simulink model "mcb_pmsm_hall_offset_f28035"  (R2021b)
settings: Solver=FixedStepDiscrete  StartTime=0.0  StopTime=Inf  RelTol=1e-3  EnableMultiTasking=on
InitFcn:
  | mcb_c2000_pmsm_offset_data;
  | target = mcb_SetProcessorDetails('F28035',PWM_frequency);
values from neighbouring files (symbols this model uses):
  PWM_frequency = 20e3    (= 20000)    [c28027pmsmfoc_data.m]    (also in c28035pmsmfoc_data.m; c28035pmsmfoc_data_cla.m = 12000; c28069pmsmfoc_data.m; mcb_c2000_open_loop_control_data.m = eval(get_param([bdroot '/Open Loop Control/Parameters/PWM Fr)
  Ts = 5e-8    (= 5e-08)    [DCDC_Buck_Param.m]    (also in mcb_c2000_open_loop_control_data.m = T_pwm; mcb_c2000_pmsm_offset_data.m = T_pwm; mcb_pmsm_foc_dual_f28379d_data.m = 5e-05; mcb_pmsm_foc_dual_f28379d_datascript.m = 5e-05)
undefined symbols (not defined in the file or in its folder): Down, GPTRIP1SEL, GPTRIP2SEL, motor, TZ1, TZ2, Up
libraries: idelinklib_common x14, simulink x5, mcbcontrolslib x5, mcbpositiondecoderlib x4, c2802xlib x4, c280xlib x3, hall_sensor_lib x3, c2803xlib x2, demo_controls x1, c2000lib x1
(part 2 of 2)

== system mcb_pmsm_hall_offset_f28035/Offset Calculation/Data Serial Output/While Iterator Subsystem ==
  Data : Inport
  Iteration : Inport  Port=2
  Add : Sum  Inputs=+-  OutDataTypeStr=Inherit: Same as first input
  Index Vector : MultiPortSwitch  Inputs=1
  SCI Transmit : c280xlib/SCI Transmit  sciModule=A  dataHead=''  dataTail=''  postInterrupt=off  numFifo=1
  While Iterator : WhileIterator  MaxIters=-1  WhileBlockType=do-while  ShowIterationPort=on  OutputDataType=int16
  wires:
  Iteration/1 -> Add/1
  Add/1 -> While Iterator/1
  Index Vector/1 -> SCI Transmit/1
  Data/1 -> Index Vector/2
  While Iterator/1 -> Index Vector/1, Add/2

== system mcb_pmsm_hall_offset_f28035/Offset Calculation/Subsystem/Calculate Position from Hall ==
  Calculate Counts : Subsystem  TreatAsAtomicUnit=on
  Data Store Read : DataStoreRead  DataStoreName=GlobalHallState  IndexOptions=Index vector (dialog)  Indices=1  OutputSizes=1
  Data Store Read2 : DataStoreRead  DataStoreName=GlobalSpeedCount  IndexOptions=Index vector (dialog)  Indices=1  OutputSizes=1
  Data Store Read3 : DataStoreRead  DataStoreName=GlobalDirection  IndexOptions=Index vector (dialog)  Indices=1  OutputSizes=1
  Data Store Read4 : DataStoreRead  DataStoreName=GlobalSpeedValidity  IndexOptions=Index vector (dialog)  Indices=1  OutputSizes=1
  Data Store Read5 : DataStoreRead  Priority=1  DataStoreName=HallStateChangeFlag  IndexOptions=Index vector (dialog)  Indices=1  OutputSizes=1
  Data Store Write2 : DataStoreWrite  Priority=2  DataStoreName=HallStateChangeFlag  IndexOptions=Index vector (dialog)  Indices=1  OutputSizes=1
  Hall Speed and Position : mcbpositiondecoderlib/Hall Speed and Position  blkExecutionType=Position  CounterSize=32 bits  ClkFreq=target.CPU_frequency  BlkSampleTime=Ts  PolePairs=motor.polePairs  MinSpeed=20  HallInterruptConfig=Every 180 Degrees  SpeedUnit=Per unit  PerUnitSpeed=6000  SpeedDataType=dataType  hallSequence=ABC  Sequence=[5,4,6,2,3,1]  EnableSecondOrder=1st Order  PositionUnit=Per unit  PositionDataType=dataType
      settings: SourceProductBaseCode=MT
  Pos_PU : Outport  InitialOutput=0  VectorParamsAs1DForOutWhenUnconnected=off
  wires:
  Hall Speed and Position/2 -> Data Store Write2/1
  Data Store Read/1 -> Calculate Counts/1(Halls), Hall Speed and Position/1
  Data Store Read5/1 -> Hall Speed and Position/6
  Data Store Read4/1 -> Hall Speed and Position/5
  Calculate Counts/1(Counter/Offset) -> Hall Speed and Position/2
  Data Store Read2/1 -> Hall Speed and Position/3
  Hall Speed and Position/1 -> Pos_PU/1
  Data Store Read3/1 -> Calculate Counts/2(Direction), Hall Speed and Position/4

== system mcb_pmsm_hall_offset_f28035/Offset Calculation/Control_System/Find Offset/Subsystem ==
  Theta_hall : Inport
  Enable : EnablePort
  IIR Filter : mcbcontrolslib/IIR Filter  VariantControl=Low Pass Filter  VariantSelect=Low-pass  Filter_constant=0.5  advancedSettings=off  Ts=50e-6  cutOff_freq=3183.0989
      settings: SourceProductBaseCode=MT
  Offset : Outport
  wires:
  IIR Filter/1 -> Offset/1
  Theta_hall/1 -> IIR Filter/1

== system mcb_pmsm_hall_offset_f28035/Offset Calculation/Control_System/PosGen/Subsystem ==
  Enable : EnablePort
  Constant : Constant  Value=0  OutDataTypeStr=Inherit: Inherit via back propagation
  Data Store Write : DataStoreWrite  DataStoreName=Enable  IndexOptions=Index vector (dialog)  Indices=1  OutputSizes=1
  wires:
  Constant/1 -> Data Store Write/1

== system mcb_pmsm_hall_offset_f28035/Offset Calculation/Control_System/PosGen/Subsystem1 ==
  Count : Inport
  Count for 2 sec : Constant  Value=2.5 * PWM_frequency  OutDataTypeStr=uint32  SampleTime=-1
  If : If  NumInputs=2  IfExpression=u1 < u2
  If Action Subsystem : Subsystem  TreatAsAtomicUnit=on
  If Action Subsystem2 : Subsystem  TreatAsAtomicUnit=on
  Merge : Merge
  Position Generator : mcbcontrolslib/Position Generator  AngleOutput=Per-unit  ThetaSource=External  ThetaInput=5e-4  DataType=double  ExternalReset=none  Offset=0
      settings: SourceProductBaseCode=MT
  Eps : Outport
  wires:
  If Action Subsystem/1(Out1) -> Merge/1
  If/1 -> If Action Subsystem/Action
  If Action Subsystem2/1(Out1) -> Merge/2
  Position Generator/1 -> Eps/1  "Eps"
  Count/1 -> If/1
  Merge/1 -> Position Generator/1
  If/2 -> If Action Subsystem2/Action
  Count for 2 sec/1 -> If/2

== system mcb_pmsm_hall_offset_f28035/Offset Calculation/Control_System/PosGen/Up Counter ==
  Enable : EnablePort  StatesWhenEnabling=reset
  Add1 : Sum  SaturateOnIntegerOverflow=on
  Constant : Constant  OutDataTypeStr=uint32
  Delay : Delay  DelayLength=1
  Count : Outport  OutputWhenDisabled=reset  InitialOutput=0
  wires:
  Add1/1 -> Count/1, Delay/1
  Constant/1 -> Add1/1
  Delay/1 -> Add1/2

== system mcb_pmsm_hall_offset_f28035/Offset Calculation/Subsystem/Calculate Position from Hall/Calculate Counts ==
  Halls : Inport
  Direction : Inport  Port=2
  Data Type Conversion2 : DataTypeConversion  OutDataTypeStr=uint32  ConvertRealWorld=Stored Integer (SI)
  Direction 0 Provides offset and counter values : Subsystem  TreatAsAtomicUnit=on
  Direction 1 Provides offset and counter values : Subsystem  TreatAsAtomicUnit=on
  Merge : Merge
  Switch on direction : If  IfExpression=u1 == 1
  Counter/Offset : Outport
  wires:
  Merge/1 -> Data Type Conversion2/1
  Switch on direction/2 -> Direction 1 Provides offset and counter values/Action
  Halls/1 -> Direction 0 Provides offset and counter values/1(halls), Direction 1 Provides offset and counter values/1(halls)
  Direction/1 -> Switch on direction/1
  Direction 0 Provides offset and counter values/1(counter) -> Merge/1
  Switch on direction/1 -> Direction 0 Provides offset and counter values/Action
  Direction 1 Provides offset and counter values/1(counter) -> Merge/2
  Data Type Conversion2/1 -> Counter/Offset/1

== system mcb_pmsm_hall_offset_f28035/Offset Calculation/Control_System/PosGen/Subsystem1/If Action Subsystem ==
  Action Port : ActionPort  ActionPortLabel=if(u1 < u2)
  Constant : Constant  Value=0  OutDataTypeStr=dataType
  Out1 : Outport
  wires:
  Constant/1 -> Out1/1

== system mcb_pmsm_hall_offset_f28035/Offset Calculation/Control_System/PosGen/Subsystem1/If Action Subsystem2 ==
  Action Port : ActionPort  ActionPortLabel=else
  Add1 : Sum
  Constant1 : Constant  Value=1e-3  OutDataTypeStr=dataType
  Delay : Delay  DelayLength=1
  Multiply : Gain  Gain=Ts  OutDataTypeStr=Inherit: Same as input
  Saturate to 60 RPM : Saturate  UpperLimit=motor.polePairs  LowerLimit=0
  Out1 : Outport
  wires:
  Delay/1 -> Add1/2
  Constant1/1 -> Add1/1
  Multiply/1 -> Out1/1
  Add1/1 -> Saturate to 60 RPM/1
  Saturate to 60 RPM/1 -> Multiply/1, Delay/1

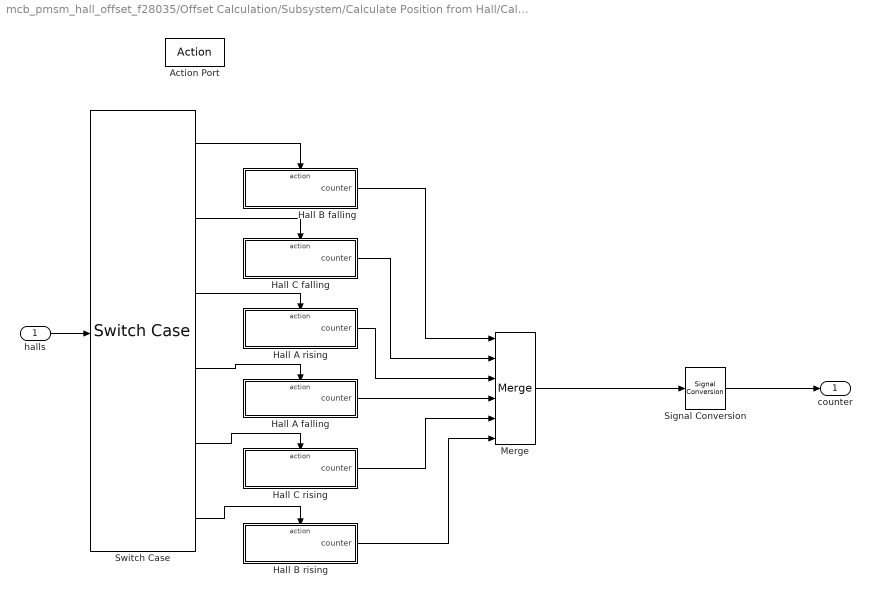
== system mcb_pmsm_hall_offset_f28035/Offset Calculation/Subsystem/Calculate Position from Hall/Calculate Counts/Direction 0 Provides offset and counter values ==
  halls : Inport
  Action Port : ActionPort
  Hall A falling : Subsystem  TreatAsAtomicUnit=on
  Hall A rising : Subsystem  TreatAsAtomicUnit=on
  Hall B falling : Subsystem  TreatAsAtomicUnit=on
  Hall B rising : Subsystem  TreatAsAtomicUnit=on
  Hall C falling : Subsystem  TreatAsAtomicUnit=on
  Hall C rising : Subsystem  TreatAsAtomicUnit=on
  Merge : Merge  Inputs=6
  Signal Conversion : SignalConversion  OverrideOpt=on
  Switch Case : SwitchCase  CaseConditions={1,2,3,4,5,6}  ShowDefaultCase=off
  counter : Outport
  wires:
  Signal Conversion/1 -> counter/1
  Hall B rising/1(counter) -> Merge/6
  Hall C rising/1(counter) -> Merge/5
  Hall A falling/1(counter) -> Merge/4
  Hall A rising/1(counter) -> Merge/3
  Hall C falling/1(counter) -> Merge/2
  Hall B falling/1(counter) -> Merge/1
  Merge/1 -> Signal Conversion/1
  Switch Case/4 -> Hall A falling/Action
  Switch Case/3 -> Hall A rising/Action
  Switch Case/1 -> Hall B falling/Action
  Switch Case/6 -> Hall B rising/Action
  Switch Case/5 -> Hall C rising/Action
  Switch Case/2 -> Hall C falling/Action
  halls/1 -> Switch Case/1

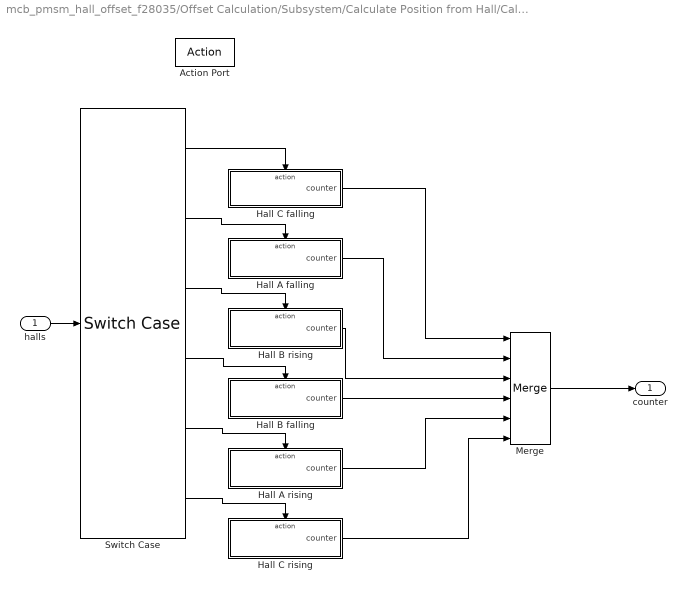
== system mcb_pmsm_hall_offset_f28035/Offset Calculation/Subsystem/Calculate Position from Hall/Calculate Counts/Direction 1 Provides offset and counter values ==
  halls : Inport
  Action Port : ActionPort
  Hall A falling : Subsystem  TreatAsAtomicUnit=on
  Hall A rising : Subsystem  TreatAsAtomicUnit=on
  Hall B falling : Subsystem  TreatAsAtomicUnit=on
  Hall B rising : Subsystem  TreatAsAtomicUnit=on
  Hall C falling : Subsystem  TreatAsAtomicUnit=on
  Hall C rising : Subsystem  TreatAsAtomicUnit=on
  Merge : Merge  Inputs=6
  Switch Case : SwitchCase  CaseConditions={1,2,3,4,5,6}  ShowDefaultCase=off
  counter : Outport
  wires:
  Hall C rising/1(counter) -> Merge/6
  Hall A rising/1(counter) -> Merge/5
  Hall B falling/1(counter) -> Merge/4
  Hall B rising/1(counter) -> Merge/3
  Hall A falling/1(counter) -> Merge/2
  Hall C falling/1(counter) -> Merge/1
  Switch Case/4 -> Hall B falling/Action
  Switch Case/3 -> Hall B rising/Action
  Switch Case/1 -> Hall C falling/Action
  Switch Case/6 -> Hall C rising/Action
  Switch Case/5 -> Hall A rising/Action
  Switch Case/2 -> Hall A falling/Action
  halls/1 -> Switch Case/1
  Merge/1 -> counter/1

== system mcb_pmsm_hall_offset_f28035/Offset Calculation/Subsystem/Calculate Position from Hall/Calculate Counts/Direction 0 Provides offset and counter values/Hall A falling ==
  Action Port : ActionPort
  ECap1Regs.TSCTR1 : idelinklib_common/Memory Copy  copyFrom=Specified source code symbol  copyFromAddressSource=Specify via dialog  copyFromAddress=hex2dec('00001000')  copyFromSrcCode=&ECap1Regs.TSCTR  dataTypeFrom=uint32  dataDimensionFrom=1  useOffsetFrom=off  offsetFromSrc=Specify via dialog  offsetFrom=0  strideFrom=1  copyTo=Output port  copyToAddressSource=Specify via dialog  copyToAddress=hex2dec('00002000')  copyToSrcCode=myVariableDst  dataTypeTo=uint32  useOffsetTo=off  offsetToSrc=Specify via dialog  offsetTo=0  strideTo=1  sampleTime=-1  useInitValue=off  initValueSrc=Specify constant value  initValue=1  initValueSrcCode=myInitValueVariable  useAsMask=off  maskOperator=bitwise AND  useTermValue=off  termValue=1  isRealtimeEnabled=off  emitCCBeforeWrite=off  CCBeforeWrite=/* Custom Code Before Write*/  emitCCAfterWrite=off  CCAfterWrite=/* Custom Code After Write*/  useDMACopy=off  enableBlockingMode=off
      settings: SourceProductBaseCode=ME
  counter : Outport
  wires:
  ECap1Regs.TSCTR1/1 -> counter/1

== system mcb_pmsm_hall_offset_f28035/Offset Calculation/Subsystem/Calculate Position from Hall/Calculate Counts/Direction 0 Provides offset and counter values/Hall A rising ==
  Action Port : ActionPort
  ECap1Regs.TSCTR1 : idelinklib_common/Memory Copy  copyFrom=Specified source code symbol  copyFromAddressSource=Specify via dialog  copyFromAddress=hex2dec('00001000')  copyFromSrcCode=&ECap1Regs.TSCTR  dataTypeFrom=uint32  dataDimensionFrom=1  useOffsetFrom=off  offsetFromSrc=Specify via dialog  offsetFrom=0  strideFrom=1  copyTo=Output port  copyToAddressSource=Specify via dialog  copyToAddress=hex2dec('00002000')  copyToSrcCode=myVariableDst  dataTypeTo=uint32  useOffsetTo=off  offsetToSrc=Specify via dialog  offsetTo=0  strideTo=1  sampleTime=-1  useInitValue=off  initValueSrc=Specify constant value  initValue=1  initValueSrcCode=myInitValueVariable  useAsMask=off  maskOperator=bitwise AND  useTermValue=off  termValue=1  isRealtimeEnabled=off  emitCCBeforeWrite=off  CCBeforeWrite=/* Custom Code Before Write*/  emitCCAfterWrite=off  CCAfterWrite=/* Custom Code After Write*/  useDMACopy=off  enableBlockingMode=off
      settings: SourceProductBaseCode=ME
  counter : Outport
  wires:
  ECap1Regs.TSCTR1/1 -> counter/1

== system mcb_pmsm_hall_offset_f28035/Offset Calculation/Subsystem/Calculate Position from Hall/Calculate Counts/Direction 0 Provides offset and counter values/Hall B falling ==
  Action Port : ActionPort
  Add : Sum  Inputs=-+  OutDataTypeStr=Inherit: Same as first input
  Data Store Read : DataStoreRead  DataStoreName=ECap1_counter_XINT1_latch  IndexOptions=Index vector (dialog)  Indices=1  OutputSizes=1
  ECap1Regs.TSCTR : idelinklib_common/Memory Copy  copyFrom=Specified source code symbol  copyFromAddressSource=Specify via dialog  copyFromAddress=hex2dec('00001000')  copyFromSrcCode=&ECap1Regs.TSCTR  dataTypeFrom=uint32  dataDimensionFrom=1  useOffsetFrom=off  offsetFromSrc=Specify via dialog  offsetFrom=0  strideFrom=1  copyTo=Output port  copyToAddressSource=Specify via dialog  copyToAddress=hex2dec('00002000')  copyToSrcCode=myVariableDst  dataTypeTo=uint32  useOffsetTo=off  offsetToSrc=Specify via dialog  offsetTo=0  strideTo=1  sampleTime=-1  useInitValue=off  initValueSrc=Specify constant value  initValue=1  initValueSrcCode=myInitValueVariable  useAsMask=off  maskOperator=bitwise AND  useTermValue=off  termValue=1  isRealtimeEnabled=off  emitCCBeforeWrite=off  CCBeforeWrite=/* Custom Code Before Write*/  emitCCAfterWrite=off  CCAfterWrite=/* Custom Code After Write*/  useDMACopy=off  enableBlockingMode=off
      settings: SourceProductBaseCode=ME
  counter : Outport
  wires:
  Add/1 -> counter/1
  ECap1Regs.TSCTR/1 -> Add/2
  Data Store Read/1 -> Add/1

== system mcb_pmsm_hall_offset_f28035/Offset Calculation/Subsystem/Calculate Position from Hall/Calculate Counts/Direction 0 Provides offset and counter values/Hall B rising ==
  Action Port : ActionPort
  Add : Sum  Inputs=-+  OutDataTypeStr=Inherit: Same as first input
  Data Store Read : DataStoreRead  DataStoreName=ECap1_counter_XINT1_latch  IndexOptions=Index vector (dialog)  Indices=1  OutputSizes=1
  ECap1Regs.TSCTR : idelinklib_common/Memory Copy  copyFrom=Specified source code symbol  copyFromAddressSource=Specify via dialog  copyFromAddress=hex2dec('00001000')  copyFromSrcCode=&ECap1Regs.TSCTR  dataTypeFrom=uint32  dataDimensionFrom=1  useOffsetFrom=off  offsetFromSrc=Specify via dialog  offsetFrom=0  strideFrom=1  copyTo=Output port  copyToAddressSource=Specify via dialog  copyToAddress=hex2dec('00002000')  copyToSrcCode=myVariableDst  dataTypeTo=uint32  useOffsetTo=off  offsetToSrc=Specify via dialog  offsetTo=0  strideTo=1  sampleTime=-1  useInitValue=off  initValueSrc=Specify constant value  initValue=1  initValueSrcCode=myInitValueVariable  useAsMask=off  maskOperator=bitwise AND  useTermValue=off  termValue=1  isRealtimeEnabled=off  emitCCBeforeWrite=off  CCBeforeWrite=/* Custom Code Before Write*/  emitCCAfterWrite=off  CCAfterWrite=/* Custom Code After Write*/  useDMACopy=off  enableBlockingMode=off
      settings: SourceProductBaseCode=ME
  counter : Outport
  wires:
  ECap1Regs.TSCTR/1 -> Add/2
  Data Store Read/1 -> Add/1
  Add/1 -> counter/1

== system mcb_pmsm_hall_offset_f28035/Offset Calculation/Subsystem/Calculate Position from Hall/Calculate Counts/Direction 0 Provides offset and counter values/Hall C falling ==
  Action Port : ActionPort
  Add : Sum  Inputs=-+  OutDataTypeStr=Inherit: Same as first input
  Data Store Read : DataStoreRead  DataStoreName=ECap1_counter_XINT2_latch  IndexOptions=Index vector (dialog)  Indices=1  OutputSizes=1
  ECap1Regs.TSCTR : idelinklib_common/Memory Copy  copyFrom=Specified source code symbol  copyFromAddressSource=Specify via dialog  copyFromAddress=hex2dec('00001000')  copyFromSrcCode=&ECap1Regs.TSCTR  dataTypeFrom=uint32  dataDimensionFrom=1  useOffsetFrom=off  offsetFromSrc=Specify via dialog  offsetFrom=0  strideFrom=1  copyTo=Output port  copyToAddressSource=Specify via dialog  copyToAddress=hex2dec('00002000')  copyToSrcCode=myVariableDst  dataTypeTo=uint32  useOffsetTo=off  offsetToSrc=Specify via dialog  offsetTo=0  strideTo=1  sampleTime=-1  useInitValue=off  initValueSrc=Specify constant value  initValue=1  initValueSrcCode=myInitValueVariable  useAsMask=off  maskOperator=bitwise AND  useTermValue=off  termValue=1  isRealtimeEnabled=off  emitCCBeforeWrite=off  CCBeforeWrite=/* Custom Code Before Write*/  emitCCAfterWrite=off  CCAfterWrite=/* Custom Code After Write*/  useDMACopy=off  enableBlockingMode=off
      settings: SourceProductBaseCode=ME
  counter : Outport
  wires:
  ECap1Regs.TSCTR/1 -> Add/2
  Data Store Read/1 -> Add/1
  Add/1 -> counter/1

== system mcb_pmsm_hall_offset_f28035/Offset Calculation/Subsystem/Calculate Position from Hall/Calculate Counts/Direction 0 Provides offset and counter values/Hall C rising ==
  Action Port : ActionPort
  Add : Sum  Inputs=-+  OutDataTypeStr=Inherit: Same as first input
  Data Store Read : DataStoreRead  DataStoreName=ECap1_counter_XINT2_latch  IndexOptions=Index vector (dialog)  Indices=1  OutputSizes=1
  ECap1Regs.TSCTR : idelinklib_common/Memory Copy  copyFrom=Specified source code symbol  copyFromAddressSource=Specify via dialog  copyFromAddress=hex2dec('00001000')  copyFromSrcCode=&ECap1Regs.TSCTR  dataTypeFrom=uint32  dataDimensionFrom=1  useOffsetFrom=off  offsetFromSrc=Specify via dialog  offsetFrom=0  strideFrom=1  copyTo=Output port  copyToAddressSource=Specify via dialog  copyToAddress=hex2dec('00002000')  copyToSrcCode=myVariableDst  dataTypeTo=uint32  useOffsetTo=off  offsetToSrc=Specify via dialog  offsetTo=0  strideTo=1  sampleTime=-1  useInitValue=off  initValueSrc=Specify constant value  initValue=1  initValueSrcCode=myInitValueVariable  useAsMask=off  maskOperator=bitwise AND  useTermValue=off  termValue=1  isRealtimeEnabled=off  emitCCBeforeWrite=off  CCBeforeWrite=/* Custom Code Before Write*/  emitCCAfterWrite=off  CCAfterWrite=/* Custom Code After Write*/  useDMACopy=off  enableBlockingMode=off
      settings: SourceProductBaseCode=ME
  counter : Outport
  wires:
  ECap1Regs.TSCTR/1 -> Add/2
  Data Store Read/1 -> Add/1
  Add/1 -> counter/1

== system mcb_pmsm_hall_offset_f28035/Offset Calculation/Subsystem/Calculate Position from Hall/Calculate Counts/Direction 1 Provides offset and counter values/Hall A falling ==
  Action Port : ActionPort
  ECap1Regs.TSCTR1 : idelinklib_common/Memory Copy  copyFrom=Specified source code symbol  copyFromAddressSource=Specify via dialog  copyFromAddress=hex2dec('00001000')  copyFromSrcCode=&ECap1Regs.TSCTR  dataTypeFrom=uint32  dataDimensionFrom=1  useOffsetFrom=off  offsetFromSrc=Specify via dialog  offsetFrom=0  strideFrom=1  copyTo=Output port  copyToAddressSource=Specify via dialog  copyToAddress=hex2dec('00002000')  copyToSrcCode=myVariableDst  dataTypeTo=uint32  useOffsetTo=off  offsetToSrc=Specify via dialog  offsetTo=0  strideTo=1  sampleTime=-1  useInitValue=off  initValueSrc=Specify constant value  initValue=1  initValueSrcCode=myInitValueVariable  useAsMask=off  maskOperator=bitwise AND  useTermValue=off  termValue=1  isRealtimeEnabled=off  emitCCBeforeWrite=off  CCBeforeWrite=/* Custom Code Before Write*/  emitCCAfterWrite=off  CCAfterWrite=/* Custom Code After Write*/  useDMACopy=off  enableBlockingMode=off
      settings: SourceProductBaseCode=ME
  counter : Outport
  wires:
  ECap1Regs.TSCTR1/1 -> counter/1

== system mcb_pmsm_hall_offset_f28035/Offset Calculation/Subsystem/Calculate Position from Hall/Calculate Counts/Direction 1 Provides offset and counter values/Hall A rising ==
  Action Port : ActionPort
  ECap1Regs.TSCTR1 : idelinklib_common/Memory Copy  copyFrom=Specified source code symbol  copyFromAddressSource=Specify via dialog  copyFromAddress=hex2dec('00001000')  copyFromSrcCode=&ECap1Regs.TSCTR  dataTypeFrom=uint32  dataDimensionFrom=1  useOffsetFrom=off  offsetFromSrc=Specify via dialog  offsetFrom=0  strideFrom=1  copyTo=Output port  copyToAddressSource=Specify via dialog  copyToAddress=hex2dec('00002000')  copyToSrcCode=myVariableDst  dataTypeTo=uint32  useOffsetTo=off  offsetToSrc=Specify via dialog  offsetTo=0  strideTo=1  sampleTime=-1  useInitValue=off  initValueSrc=Specify constant value  initValue=1  initValueSrcCode=myInitValueVariable  useAsMask=off  maskOperator=bitwise AND  useTermValue=off  termValue=1  isRealtimeEnabled=off  emitCCBeforeWrite=off  CCBeforeWrite=/* Custom Code Before Write*/  emitCCAfterWrite=off  CCAfterWrite=/* Custom Code After Write*/  useDMACopy=off  enableBlockingMode=off
      settings: SourceProductBaseCode=ME
  counter : Outport
  wires:
  ECap1Regs.TSCTR1/1 -> counter/1

== system mcb_pmsm_hall_offset_f28035/Offset Calculation/Subsystem/Calculate Position from Hall/Calculate Counts/Direction 1 Provides offset and counter values/Hall B falling ==
  Action Port : ActionPort
  Add : Sum  Inputs=+-  OutDataTypeStr=Inherit: Same as first input
  Data Store Read : DataStoreRead  DataStoreName=ECap1_counter_XINT1_latch  IndexOptions=Index vector (dialog)  Indices=1  OutputSizes=1
  ECap1Regs.TSCTR : idelinklib_common/Memory Copy  copyFrom=Specified source code symbol  copyFromAddressSource=Specify via dialog  copyFromAddress=hex2dec('00001000')  copyFromSrcCode=&ECap1Regs.TSCTR  dataTypeFrom=uint32  dataDimensionFrom=1  useOffsetFrom=off  offsetFromSrc=Specify via dialog  offsetFrom=0  strideFrom=1  copyTo=Output port  copyToAddressSource=Specify via dialog  copyToAddress=hex2dec('00002000')  copyToSrcCode=myVariableDst  dataTypeTo=uint32  useOffsetTo=off  offsetToSrc=Specify via dialog  offsetTo=0  strideTo=1  sampleTime=-1  useInitValue=off  initValueSrc=Specify constant value  initValue=1  initValueSrcCode=myInitValueVariable  useAsMask=off  maskOperator=bitwise AND  useTermValue=off  termValue=1  isRealtimeEnabled=off  emitCCBeforeWrite=off  CCBeforeWrite=/* Custom Code Before Write*/  emitCCAfterWrite=off  CCAfterWrite=/* Custom Code After Write*/  useDMACopy=off  enableBlockingMode=off
      settings: SourceProductBaseCode=ME
  counter : Outport
  wires:
  ECap1Regs.TSCTR/1 -> Add/1
  Data Store Read/1 -> Add/2
  Add/1 -> counter/1

== system mcb_pmsm_hall_offset_f28035/Offset Calculation/Subsystem/Calculate Position from Hall/Calculate Counts/Direction 1 Provides offset and counter values/Hall B rising ==
  Action Port : ActionPort
  Add : Sum  Inputs=-+  OutDataTypeStr=Inherit: Same as first input
  Data Store Read : DataStoreRead  DataStoreName=ECap1_counter_XINT1_latch  IndexOptions=Index vector (dialog)  Indices=1  OutputSizes=1
  ECap1Regs.TSCTR : idelinklib_common/Memory Copy  copyFrom=Specified source code symbol  copyFromAddressSource=Specify via dialog  copyFromAddress=hex2dec('00001000')  copyFromSrcCode=&ECap1Regs.TSCTR  dataTypeFrom=uint32  dataDimensionFrom=1  useOffsetFrom=off  offsetFromSrc=Specify via dialog  offsetFrom=0  strideFrom=1  copyTo=Output port  copyToAddressSource=Specify via dialog  copyToAddress=hex2dec('00002000')  copyToSrcCode=myVariableDst  dataTypeTo=uint32  useOffsetTo=off  offsetToSrc=Specify via dialog  offsetTo=0  strideTo=1  sampleTime=-1  useInitValue=off  initValueSrc=Specify constant value  initValue=1  initValueSrcCode=myInitValueVariable  useAsMask=off  maskOperator=bitwise AND  useTermValue=off  termValue=1  isRealtimeEnabled=off  emitCCBeforeWrite=off  CCBeforeWrite=/* Custom Code Before Write*/  emitCCAfterWrite=off  CCAfterWrite=/* Custom Code After Write*/  useDMACopy=off  enableBlockingMode=off
      settings: SourceProductBaseCode=ME
  counter : Outport
  wires:
  ECap1Regs.TSCTR/1 -> Add/2
  Data Store Read/1 -> Add/1
  Add/1 -> counter/1

== system mcb_pmsm_hall_offset_f28035/Offset Calculation/Subsystem/Calculate Position from Hall/Calculate Counts/Direction 1 Provides offset and counter values/Hall C falling ==
  Action Port : ActionPort
  Add : Sum  Inputs=-+  OutDataTypeStr=Inherit: Same as first input
  Data Store Read : DataStoreRead  DataStoreName=ECap1_counter_XINT2_latch  IndexOptions=Index vector (dialog)  Indices=1  OutputSizes=1
  ECap1Regs.TSCTR : idelinklib_common/Memory Copy  copyFrom=Specified source code symbol  copyFromAddressSource=Specify via dialog  copyFromAddress=hex2dec('00001000')  copyFromSrcCode=&ECap1Regs.TSCTR  dataTypeFrom=uint32  dataDimensionFrom=1  useOffsetFrom=off  offsetFromSrc=Specify via dialog  offsetFrom=0  strideFrom=1  copyTo=Output port  copyToAddressSource=Specify via dialog  copyToAddress=hex2dec('00002000')  copyToSrcCode=myVariableDst  dataTypeTo=uint32  useOffsetTo=off  offsetToSrc=Specify via dialog  offsetTo=0  strideTo=1  sampleTime=-1  useInitValue=off  initValueSrc=Specify constant value  initValue=1  initValueSrcCode=myInitValueVariable  useAsMask=off  maskOperator=bitwise AND  useTermValue=off  termValue=1  isRealtimeEnabled=off  emitCCBeforeWrite=off  CCBeforeWrite=/* Custom Code Before Write*/  emitCCAfterWrite=off  CCAfterWrite=/* Custom Code After Write*/  useDMACopy=off  enableBlockingMode=off
      settings: SourceProductBaseCode=ME
  counter : Outport
  wires:
  Data Store Read/1 -> Add/1
  ECap1Regs.TSCTR/1 -> Add/2
  Add/1 -> counter/1

== system mcb_pmsm_hall_offset_f28035/Offset Calculation/Subsystem/Calculate Position from Hall/Calculate Counts/Direction 1 Provides offset and counter values/Hall C rising ==
  Action Port : ActionPort
  Add : Sum  Inputs=-+  OutDataTypeStr=Inherit: Same as first input
  Data Store Read : DataStoreRead  DataStoreName=ECap1_counter_XINT2_latch  IndexOptions=Index vector (dialog)  Indices=1  OutputSizes=1
  ECap1Regs.TSCTR : idelinklib_common/Memory Copy  copyFrom=Specified source code symbol  copyFromAddressSource=Specify via dialog  copyFromAddress=hex2dec('00001000')  copyFromSrcCode=&ECap1Regs.TSCTR  dataTypeFrom=uint32  dataDimensionFrom=1  useOffsetFrom=off  offsetFromSrc=Specify via dialog  offsetFrom=0  strideFrom=1  copyTo=Output port  copyToAddressSource=Specify via dialog  copyToAddress=hex2dec('00002000')  copyToSrcCode=myVariableDst  dataTypeTo=uint32  useOffsetTo=off  offsetToSrc=Specify via dialog  offsetTo=0  strideTo=1  sampleTime=-1  useInitValue=off  initValueSrc=Specify constant value  initValue=1  initValueSrcCode=myInitValueVariable  useAsMask=off  maskOperator=bitwise AND  useTermValue=off  termValue=1  isRealtimeEnabled=off  emitCCBeforeWrite=off  CCBeforeWrite=/* Custom Code Before Write*/  emitCCAfterWrite=off  CCAfterWrite=/* Custom Code After Write*/  useDMACopy=off  enableBlockingMode=off
      settings: SourceProductBaseCode=ME
  counter : Outport
  wires:
  Data Store Read/1 -> Add/1
  ECap1Regs.TSCTR/1 -> Add/2
  Add/1 -> counter/1
